simulink model "arch_logical"  (R2026a)
settings: Solver=daessc  MaxStep=MCU_Ts_FOC  RelTol=0.01
undefined symbols (not defined in the file): MCU_Ts_FOC, Param_SigProcessing_SpeedMeas_Delays, Req_Caps_Motor_Currents, Req_Caps_Motor_Torques, Req_Caps_Motor_Velocity, Req_Caps_Transmission_Torques, Req_Caps_Transmission_Velocity
libraries: simulink x5, mcbpositiondecoderlib x1
(part 2 of 2)

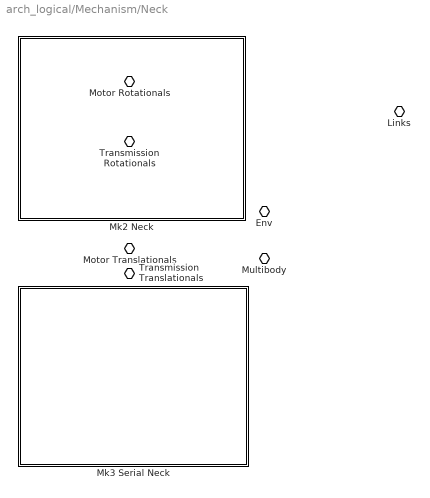
== system arch_logical/Mechanism/Neck ==
  Mk2 Neck : Subsystem  VariantControl=Selector_Mechanism == Types_Mechanism.Mk2  ReferencedSubsystem=Mk2NeckWrapper
      settings: PermitHierarchicalResolution=None  PortSchema="{\"entries\":[{\"content\":{\"headerSize\":26,\"margin\":15,\"minimumSpacing\":25,\"sides\":[{\"content\":{\"connectorIds\":[\"LConn1\",\"LConn2\"]},\"type\":\"ConnectorPlacement.EquallySpacedRectSide\",\"uuid\":\"57d6c408-3008-4772-82fa-c78950aeb972\"},{\"content\":{\"connectorIds\":[\"RConn2\"],\"side\":\"RIGHT\"},\"type\":\"ConnectorPlacement.EquallySpacedRectSide\",\"uuid\":\"be30f5ae-b864-4f0d-80fa-3961a8cb329f\"},{\"content\":{\"side\":\"TOP\"},\"type\":\"ConnectorPlacement.EquallySpacedRectSide\",\"uuid\":\"34d93d68-430e-44f9-8eee-ecae2c4e1418\"},{\"content\":{\"connectorIds\":[\"RConn1\",\"RConn3\"],\"side\":\"BOTTOM\"},\"type\":\"ConnectorPlacement.EquallySpacedRectSide\",\"uuid\":\"c172c7ca-a849-4a61-b14b-b119063e659c\"}]},\"type\":\"ConnectorPlacement.EquallySpacedConnector\",\"uuid\":\"47a4edbe-a09b-4305-8f4f-fa3fc9056d60\"}],\"packageUris\":[\"http://schema.mathworks.com/mf0/Connector/R2020b\"],\"version\":\"1.0\"}"
  Mk3 Serial Neck : Subsystem  VariantControl=Selector_Mechanism == Types_Mechanism.Mk3_Serial  ReferencedSubsystem=Mk3SerialNeckWrapper
      settings: PermitHierarchicalResolution=None  PortSchema="{\"entries\":[{\"content\":{\"headerSize\":26,\"margin\":15,\"minimumSpacing\":25,\"sides\":[{\"content\":{\"connectorIds\":[\"LConn1\"]},\"type\":\"ConnectorPlacement.EquallySpacedRectSide\",\"uuid\":\"25b65f7d-f824-4ba3-b1ed-62665898e2af\"},{\"content\":{\"connectorIds\":[\"RConn2\"],\"side\":\"RIGHT\"},\"type\":\"ConnectorPlacement.EquallySpacedRectSide\",\"uuid\":\"9487a21d-3ba6-4fe2-bdba-f10d1b29e9d5\"},{\"content\":{\"side\":\"TOP\"},\"type\":\"ConnectorPlacement.EquallySpacedRectSide\",\"uuid\":\"4746a095-1b27-40e2-b199-adb40e90c46e\"},{\"content\":{\"connectorIds\":[\"RConn1\",\"RConn3\"],\"side\":\"BOTTOM\"},\"type\":\"ConnectorPlacement.EquallySpacedRectSide\",\"uuid\":\"8bc943fb-2130-466d-ab3f-feb20f26c439\"}]},\"type\":\"ConnectorPlacement.EquallySpacedConnector\",\"uuid\":\"2d26b106-d6e1-4bff-b1c2-31dab5640331\"}],\"packageUris\":[\"http://schema.mathworks.com/mf0/Connector/R2020b\"],\"version\":\"1.0\"}"
  Motor Rotationals : PMIOPort  Side=Left  ConnectionType=Bus: Physical_MotorRotationals
  Motor Translationals : PMIOPort  Port=2  Side=Left  ConnectionType=Bus: Physical_MotorTranslationals
  Transmission Rotationals : PMIOPort  Port=3  Side=Left  ConnectionType=Bus: Physical_TransmissionRotationals
  Links : PMIOPort  Port=4  Side=Right
  Multibody : PMIOPort  Port=5  Side=Right  ConnectionType=Bus: Physical_Multibody
  Env : PMIOPort  Port=6  Side=Right  ConnectionType=Bus: Physical_Environment
  Transmission Translationals : PMIOPort  Port=7  Side=Left  ConnectionType=Bus: Physical_TransmissionTranslationals

== system arch_logical/Mechanism/Payload ==
  ergoCub Head : Subsystem  VariantControl=Selector_Payload == Types_Payload.ergoCubHead  ReferencedSubsystem=ergoCubHeadWrapper
      settings: PermitHierarchicalResolution=None  PortSchema="{\"entries\":[{\"content\":{\"headerSize\":26,\"margin\":15,\"minimumSpacing\":25,\"sides\":[{\"content\":{\"connectorIds\":[\"LConn1\"]},\"type\":\"ConnectorPlacement.EquallySpacedRectSide\",\"uuid\":\"57d6c408-3008-4772-82fa-c78950aeb972\"},{\"content\":{\"side\":\"RIGHT\"},\"type\":\"ConnectorPlacement.EquallySpacedRectSide\",\"uuid\":\"be30f5ae-b864-4f0d-80fa-3961a8cb329f\"},{\"content\":{\"side\":\"TOP\"},\"type\":\"ConnectorPlacement.EquallySpacedRectSide\",\"uuid\":\"34d93d68-430e-44f9-8eee-ecae2c4e1418\"}]},\"type\":\"ConnectorPlacement.EquallySpacedConnector\",\"uuid\":\"47a4edbe-a09b-4305-8f4f-fa3fc9056d60\"}],\"packageUris\":[\"http://schema.mathworks.com/mf0/Connector/R2020b\"],\"version\":\"1.0\"}"
  ergoCub Head with Eyes : Subsystem  VariantControl=Selector_Payload == Types_Payload.ergoCubHeadWithEyes  ReferencedSubsystem=ergoCubHeadWithEyesWrapper
      settings: PermitHierarchicalResolution=None  PortSchema="{\"entries\":[{\"content\":{\"headerSize\":26,\"margin\":15,\"minimumSpacing\":25,\"sides\":[{\"content\":{\"connectorIds\":[\"LConn1\"]},\"type\":\"ConnectorPlacement.EquallySpacedRectSide\",\"uuid\":\"fc112f56-f4f6-4444-b2ad-6908f72a4311\"},{\"content\":{\"side\":\"RIGHT\"},\"type\":\"ConnectorPlacement.EquallySpacedRectSide\",\"uuid\":\"d676f033-1cf0-4c6e-9277-6d5c9fd14db0\"},{\"content\":{\"side\":\"TOP\"},\"type\":\"ConnectorPlacement.EquallySpacedRectSide\",\"uuid\":\"9d93c446-f455-42a3-850a-2221f29f819d\"}]},\"type\":\"ConnectorPlacement.EquallySpacedConnector\",\"uuid\":\"8bf59047-f665-4089-9fec-3c3cb04693b3\"}],\"packageUris\":[\"http://schema.mathworks.com/mf0/Connector/R2020b\"],\"version\":\"1.0\"}"
  iCub Head : Subsystem  VariantControl=Selector_Payload == Types_Payload.iCubHead  ReferencedSubsystem=iCubHeadWrapper
      settings: PermitHierarchicalResolution=None  PortSchema="{\"entries\":[{\"content\":{\"headerSize\":26,\"margin\":15,\"minimumSpacing\":25,\"sides\":[{\"content\":{\"connectorIds\":[\"LConn1\"]},\"type\":\"ConnectorPlacement.EquallySpacedRectSide\",\"uuid\":\"94711968-37c4-489b-b3a5-96fb511461b1\"},{\"content\":{\"side\":\"RIGHT\"},\"type\":\"ConnectorPlacement.EquallySpacedRectSide\",\"uuid\":\"a2df9540-f21c-412c-a79a-61aea4ce4494\"},{\"content\":{\"side\":\"TOP\"},\"type\":\"ConnectorPlacement.EquallySpacedRectSide\",\"uuid\":\"2c7f32cd-83c4-44ef-9861-d2cdf3ae6cf3\"}]},\"type\":\"ConnectorPlacement.EquallySpacedConnector\",\"uuid\":\"5180f687-85a7-44b2-831d-1412b0c572e8\"}],\"packageUris\":[\"http://schema.mathworks.com/mf0/Connector/R2020b\"],\"version\":\"1.0\"}"
  Links : PMIOPort  Side=Left

== system arch_logical/Sensing/Impairments ==
  Measurements In : Inport  OutDataTypeStr=Bus: Data_Measurements
  Ideal : Subsystem  VariantControl=Selector_Impairments == Types_Impairments.Ideal
      settings: PortSchema="{\"entries\":[{\"content\":{\"headerSize\":26,\"margin\":15,\"minimumSpacing\":25,\"sides\":[{\"content\":{\"connectorIds\":[\"Out1\"]},\"type\":\"ConnectorPlacement.EquallySpacedRectSide\",\"uuid\":\"adb94743-de46-43b3-8f5b-4e3d902d46b9\"},{\"content\":{\"connectorIds\":[\"In1\"],\"side\":\"RIGHT\"},\"type\":\"ConnectorPlacement.EquallySpacedRectSide\",\"uuid\":\"3d40f326-48c5-47c9-b6f5-5e68818bd70e\"},{\"content\":{\"side\":\"TOP\"},\"type\":\"ConnectorPlacement.EquallySpacedRectSide\",\"uuid\":\"35996a1f-7231-45c6-9398-88da53b9d412\"}]},\"type\":\"ConnectorPlacement.EquallySpacedConnector\",\"uuid\":\"901aa676-84bd-40f0-a38d-8b9c20d85e30\"}],\"packageUris\":[\"http://schema.mathworks.com/mf0/Connector/R2020b\"],\"version\":\"1.0\"}"
  Mk3 Serial Impairments : Subsystem  VariantControl=Selector_Impairments == Types_Impairments.Mk3_Serial  ReferencedSubsystem=Mk3SerialImpairments
      settings: PermitHierarchicalResolution=None  PortSchema="{\"entries\":[{\"content\":{\"headerSize\":26,\"margin\":15,\"minimumSpacing\":25,\"sides\":[{\"content\":{\"connectorIds\":[\"Out1\"]},\"type\":\"ConnectorPlacement.EquallySpacedRectSide\",\"uuid\":\"49c15c88-294a-49d3-a3e9-7e9d2d7e0fbb\"},{\"content\":{\"connectorIds\":[\"In1\"],\"side\":\"RIGHT\"},\"type\":\"ConnectorPlacement.EquallySpacedRectSide\",\"uuid\":\"231f3a62-e970-4c5e-be8a-7dda6d603d83\"},{\"content\":{\"side\":\"TOP\"},\"type\":\"ConnectorPlacement.EquallySpacedRectSide\",\"uuid\":\"403ac151-60ed-4891-8e31-1a38c9d325e1\"}]},\"type\":\"ConnectorPlacement.EquallySpacedConnector\",\"uuid\":\"3d0f34fd-30d8-4e40-9b1c-23769127a566\"}],\"packageUris\":[\"http://schema.mathworks.com/mf0/Connector/R2020b\"],\"version\":\"1.0\"}"
  Measurements Out : Outport  OutDataTypeStr=Bus: Data_Measurements

== system arch_logical/MCU/Planner/Planner None ==
  Bus Element In1 : Inport  PortName=Joint References In
  Bus Element Out1 : Outport  PortName=Joint References Out
  wires:
  Bus Element In1/1 -> Bus Element Out1/1

== system arch_logical/MCU/Signal Processing/Signal Processing None ==
  Bus Element In1 : Inport  PortName=Measurements
  Bus Creator : BusCreator  Inputs=3  OutDataTypeStr=Bus: Data_ControlFeedback  NonVirtualBus=on
      settings: InheritFromInputs=off
  Bus Selector : BusSelector  OutputSignals=Encoders,Currents
  Speed Measurement : mcbpositiondecoderlib/Speed Measurement  DiscreteStepInput=off  LastDiscreteStepInput=off  PositionUnit=Degrees  PositionScalingDatatype=uint32  SpeedCalculationMode=Time interval for speed calculation  TempSpeedCalculationMode=Time interval for speed calculation  SampleTimeAsync=MCU_Ts  MaximumApplicationSpeed=1000  SpeedResolution=10^-5/6  DelayLength=Param_SigProcessing_SpeedMeas_Delays  MaximumMeasurableSpeed=6000  MeasurableSpeedResolution=3.4925e-06  SpeedUnit=Degrees/Sec  TempSpeedUnit=RPM  PerUnitSpeed=1000  SpeedDataType=single
      settings: LibrarySourceBlock=mcblib/Sensor Decoders/Speed Measurement
  Bus Element Out1 : Outport  PortName=Control Feedback
  wires:
  Bus Element In1/1 -> Bus Selector/1
  Bus Creator/1 -> Bus Element Out1/1
  Bus Selector/1 -> Speed Measurement/1, Bus Creator/1  "<Encoders>"
  Bus Selector/2 -> Bus Creator/3  "<Currents>"
  Speed Measurement/1 -> Bus Creator/2

== system arch_logical/Sensing/Impairments/Ideal ==
  Bus Element In2 : Inport  PortName=Measurements In
  Bus Element Out1 : Outport  PortName=Measurements Out
  wires:
  Bus Element In2/1 -> Bus Element Out1/1
